simulink model "up3control"  (R2017b)
settings: Solver=FixedStepAuto  StartTime=0.0  StopTime=15  FixedStep=1e-3  RelTol=1e-6
values from neighbouring files (symbols this model uses):
  g = 9.80    (= 9.8)    [calcSystem.m]    (also in sysNonlinearSfunc.m)
  I = 1/3*m*l^2    (= 0.00227083333333)    [calcSystem.m]    (also in sysNonlinearSfunc.m = block.DialogPrm(5).Data)
  Klqr3 = designLQR(A2, B2, diag([900,0,100,0]), 1)    [calcSystem.m]
  l = 0.25    [calcSystem.m]    (also in sysNonlinearSfunc.m = block.DialogPrm(4).Data)
  m = 0.109    [calcSystem.m]    (also in sysNonlinearSfunc.m = block.DialogPrm(2).Data)
settings Model: Creator=Haotian  LastModifiedBy=Haotian

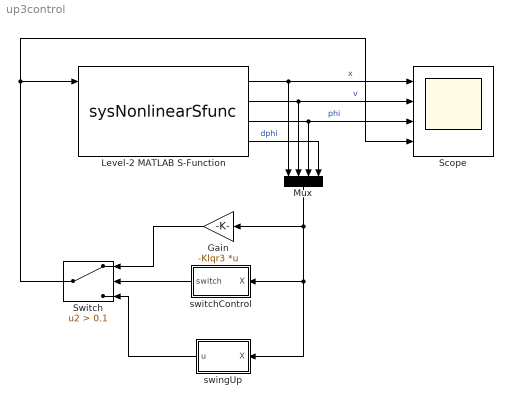
== system up3control ==
  Gain : Gain  Gain=-Klqr3  Multiplication=Matrix(K*u)
  Level-2 MATLAB S-Function : M-S-Function  FunctionName=sysNonlinearSfunc  Parameters=Mc, Mg, b, l, I, init_phi, useAcc  mask(S-function: sysNonlinearSfunc){Mc=1.096, Mg=0.109, b=0.1, l=0.25, I=0.0025, init_phi=pi - 0.01, useAcc=on}
      mask prompts: Mc "小车质量"; Mg "摆杆质量"; b "小车摩擦系数"; l "摆杆转动轴心到杆质心的长度"; I "摆杆惯量"; init_phi "初始垂直夹角"; useAcc "使用加速度作为输入"
      mask help: 一阶倒立摆非线性模型。
      mask Display:
      | fprintf('一阶倒立摆\n\nM=%.3f m=%.3f\nb=%.3f l=%.3f\nI=%.3f phi0=%.2f\n\nX=[x dx phi dphi]', Mc, Mg, b, l, I, init_phi);
      | if(useAcc)
      |     port_label('input', 1, 'a');
      | else
      |     port_label('input', 1, 'F');
      | end
      | port_label('input', 2, 'setX');
      | port_label('input', 3, 'devX');
      | 
      | port_label('output', 1, 'x');
      | port_label('output', 2, 'v');
      | port_label('output', 3, '\phi','texmode','on');
      | port_label('output', 4, 'd\phi','texmode','on');
  Mux : Mux
  Scope : Scope  NumInputPorts=4
  Switch : Switch  Criteria=u2 > Threshold  Threshold=0.1
  swingUp : Subsystem
  switchControl : Subsystem
  wires:
  Switch/1 -> Scope/4, Level-2 MATLAB S-Function/1
  Level-2 MATLAB S-Function/1 -> Mux/1, Scope/1  "x"
  Level-2 MATLAB S-Function/3 -> Scope/3, Mux/3  "phi"
  Gain/1 -> Switch/1
  switchControl/1(switch) -> Switch/2
  Level-2 MATLAB S-Function/4 -> Mux/4  "dphi"
  Mux/1 -> switchControl/1(X), swingUp/1(X), Gain/1
  Level-2 MATLAB S-Function/2 -> Scope/2, Mux/2  "v"
  swingUp/1(u) -> Switch/3

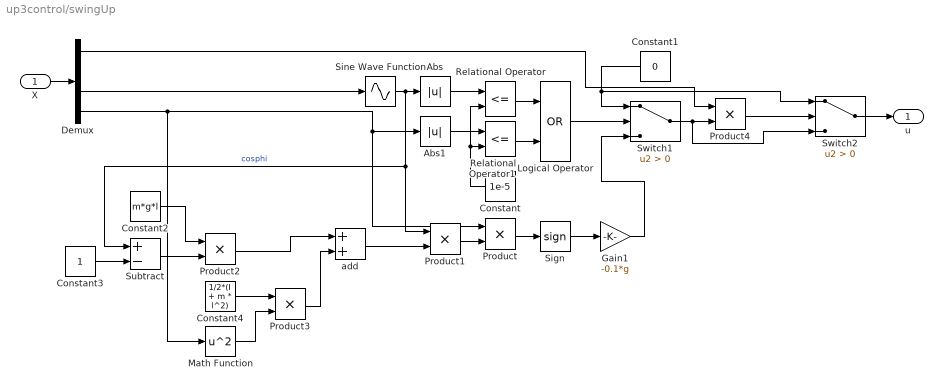
== system up3control/swingUp ==
  X : Inport
  Abs : Abs
  Abs1 : Abs
  Constant : Constant  Value=1e-5
  Constant1 : Constant  Value=0
  Constant2 : Constant  Value=m*g*l
  Constant3 : Constant
  Constant4 : Constant  Value=1/2*(I + m * l^2)
  Demux : Demux
  Gain1 : Gain  Gain=-0.1*g
  Logical Operator : Logic  Operator=OR  AllPortsSameDT=off  OutDataTypeStr=boolean
  Math Function : Math  Operator=square  SaturateOnIntegerOverflow=on
  Product{,1..4} (5 alike) : Product
  Relational Operator : RelationalOperator  Operator=<=  OutDataTypeStr=boolean  RndMeth=Simplest
  Relational Operator1 : RelationalOperator  Operator=<=  OutDataTypeStr=boolean  RndMeth=Simplest
  Sign : Signum
  Sine Wave Function : Sin  TimeSource=Use external signal  Phase=pi/2  SampleTime=0
  Subtract : Sum  Inputs=+-
  Switch1 : Switch  Criteria=u2 > Threshold
  Switch2 : Switch  Criteria=u2 > Threshold
  add : Sum
  u : Outport
  wires:
  Product2/1 -> add/1
  Constant3/1 -> Subtract/2
  Abs/1 -> Relational Operator/1
  Relational Operator1/1 -> Logical Operator/2
  Relational Operator/1 -> Logical Operator/1
  Constant/1 -> Relational Operator1/2, Relational Operator/2
  Subtract/1 -> Product2/2
  Product3/1 -> add/2
  Logical Operator/1 -> Switch1/2
  Abs1/1 -> Relational Operator1/1
  Product1/1 -> Product/2
  Product/1 -> Sign/1
  add/1 -> Product1/2
  Constant1/1 -> Switch2/1, Switch1/1
  Constant4/1 -> Product3/1
  Sign/1 -> Gain1/1
  Product4/1 -> Switch2/2
  Gain1/1 -> Switch1/3
  Demux/1 -> Product4/1
  Switch1/1 -> Switch2/3, Product4/2
  Demux/4 -> Math Function/1, Abs1/1, Product/1
  Sine Wave Function/1 -> Subtract/1, Product1/1, Abs/1  "cosphi"
  Demux/3 -> Sine Wave Function/1
  Switch2/1 -> u/1
  X/1 -> Demux/1
  Math Function/1 -> Product3/2
  Constant2/1 -> Product2/1

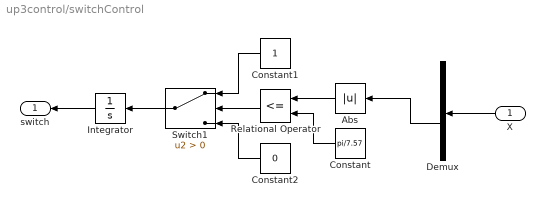
== system up3control/switchControl ==
  X : Inport
  Abs : Abs
  Constant : Constant  Value=pi/7.57
  Constant1 : Constant
  Constant2 : Constant  Value=0
  Demux : Demux
  Integrator : Integrator
  Relational Operator : RelationalOperator  Operator=<=  OutDataTypeStr=boolean  RndMeth=Simplest
  Switch1 : Switch  Criteria=u2 > Threshold
  switch : Outport
  wires:
  Constant2/1 -> Switch1/3
  Demux/3 -> Abs/1
  X/1 -> Demux/1
  Switch1/1 -> Integrator/1
  Constant/1 -> Relational Operator/2
  Constant1/1 -> Switch1/1
  Abs/1 -> Relational Operator/1
  Relational Operator/1 -> Switch1/2
  Integrator/1 -> switch/1
